simulink model "System3"  (R2025a)
settings: Solver=ode113  StartTime=0.0  StopTime=400  FixedStep=0.01  MaxStep=0.1  RelTol=1e-3
libraries: simulink x3784, slpidlib x2
(part 91 of 160)

== system System3/Battery1/Module3/SubModule_10/Cell9/SOC_Mapping ==
  SOC : Inport
  Cell_Temp : Inport  Port=2
  2-D Lookup Table : Lookup_n-D  LookupTableObject=''  BreakpointsForDimension1Source=Input port  BreakpointsForDimension1=[0 0.1 0.2 0.3 0.4 0.5 0.6 0.7 0.8 0.9 1]  BreakpointsForDimension2=[0 10 20 30 40 50 60]  BreakpointsForDimension1FirstPoint=10  BreakpointsForDimension2FirstPoint=10  BreakpointsForDimension1Spacing=12  BreakpointsForDimension2Spacing=12  IndexSearchMethod=Evenly spaced points  TableSource=Input port  Table=|  InterpMethod=Akima spline  DiagnosticForOutOfRangeInput=Error  InternalRulePriority=Speed  RndMeth=Simplest
      | [
      |     2.954364, 3.109857, 3.273534, 3.3066, 3.34,    3.3734,  3.20473;
      |     3.122427, 3.286765, 3.459753, 3.4947, 3.53,    3.5653,  3.387035;
      |     3.175499, 3.342631, 3.518559, 3.5541, 3.59,    3.6259,  3.444605;
      |     3.210881, 3.379875, 3.557763, 3.5937, 3.63,    3.6663,  3.482985;
      |     3.237417, 3.407808, 3.587166, 3.6234, 3.66,    3.6966,  3.511777;
      |     3.272799, 3.445052, 3.62637,  3.663,  3.7,     3.737,   3.55015;
      |     3.317026, 3.491066, 3.675375, 3.7125, 3.75,    3.7875,  3.598125;
      |     3.387789, 3.566094, 3.753783, 3.7917, 3.83,    3.8683,  3.674885;
      |     3.467398, 3.649892, 3.841992, 3.8808, 3.92,    3.9592,  3.76124;
      |     3.564697, 3.752313, 3.949803, 3.9897, 4.03,    4.0703,  3.866785;
      |     3.653151, 3.845422, 4.047813, 4.0887, 4.13,    4.1713,  3.962735
      | ]
      settings: InputPortMap=u0,u1,p221,p5
  2-D Lookup Table1 : Lookup_n-D  LookupTableObject=''  BreakpointsForDimension1Source=Input port  BreakpointsForDimension1=[0 0.1 0.2 0.3 0.4 0.5 0.6 0.7 0.8 0.9 1]  BreakpointsForDimension2=[0 10 20 30 40 50 60]  BreakpointsForDimension1FirstPoint=10  BreakpointsForDimension2FirstPoint=10  BreakpointsForDimension1Spacing=12  BreakpointsForDimension2Spacing=12  IndexSearchMethod=Evenly spaced points  TableSource=Input port  Table=|  InterpMethod=Akima spline  DiagnosticForOutOfRangeInput=Error  InternalRulePriority=Speed  RndMeth=Simplest
      | [
      |     2.954364, 3.109857, 3.273534, 3.3066, 3.34,    3.3734,  3.20473;
      |     3.122427, 3.286765, 3.459753, 3.4947, 3.53,    3.5653,  3.387035;
      |     3.175499, 3.342631, 3.518559, 3.5541, 3.59,    3.6259,  3.444605;
      |     3.210881, 3.379875, 3.557763, 3.5937, 3.63,    3.6663,  3.482985;
      |     3.237417, 3.407808, 3.587166, 3.6234, 3.66,    3.6966,  3.511777;
      |     3.272799, 3.445052, 3.62637,  3.663,  3.7,     3.737,   3.55015;
      |     3.317026, 3.491066, 3.675375, 3.7125, 3.75,    3.7875,  3.598125;
      |     3.387789, 3.566094, 3.753783, 3.7917, 3.83,    3.8683,  3.674885;
      |     3.467398, 3.649892, 3.841992, 3.8808, 3.92,    3.9592,  3.76124;
      |     3.564697, 3.752313, 3.949803, 3.9897, 4.03,    4.0703,  3.866785;
      |     3.653151, 3.845422, 4.047813, 4.0887, 4.13,    4.1713,  3.962735
      | ]
      settings: InputPortMap=u0,u1,p221,p5
  Lookup Table Dynamic{3..6} (4 alike) : simulink/Lookup Tables/Lookup Table Dynamic  LookUpMeth=Interpolation-Use End Values  OutDataType=fixdt('double')  OutScaling=[]  OutputDataTypeScalingMode=Specify via dialog  OutDataTypeStr=fixdt('double')  DoSatur=off
  Ri : Outport
  R1 : Outport  Port=2
  C1 : Outport  Port=3
  R2 : Outport  Port=4
  C2 : Outport  Port=5
  OCV : Outport  Port=6
  wires:
  SOC/1 -> Lookup Table Dynamic3/1, Lookup Table Dynamic6/1, Lookup Table Dynamic5/1, Lookup Table Dynamic4/1, 2-D Lookup Table1/1, 2-D Lookup Table/1
  [SOC_User] -> 2-D Lookup Table/4, Lookup Table Dynamic6/2, Lookup Table Dynamic5/2, Lookup Table Dynamic4/2, Lookup Table Dynamic3/2, 2-D Lookup Table1/4
  [OCV] -> 2-D Lookup Table/3
  2-D Lookup Table/1 -> OCV/1
  [Ri_User] -> 2-D Lookup Table1/3
  2-D Lookup Table1/1 -> Ri/1
  [R1_User] -> Lookup Table Dynamic3/3
  Lookup Table Dynamic3/1 -> R1/1
  [C1_User] -> Lookup Table Dynamic4/3
  Lookup Table Dynamic4/1 -> C1/1
  [R2_User] -> Lookup Table Dynamic5/3
  Lookup Table Dynamic5/1 -> R2/1
  [C2_User] -> Lookup Table Dynamic6/3
  Lookup Table Dynamic6/1 -> C2/1
  Cell_Temp/1 -> 2-D Lookup Table1/2, 2-D Lookup Table/2

== system System3/Battery1/Module3/SubModule_10/Cell9/Subsystem ==
  Cell_Current : Inport
  Ri : Inport  Port=2
  Add : Sum  Inputs=+-
  Add1 : Sum  Inputs=-+
  Delay : Delay  DelayLength=1  InitialConditionSource=Input port
      settings: InputPortMap=u0,p4
  Divide : Product  Inputs=*/
  From3 : From  TagVisibility=global
  Integrator : Integrator  InitialConditionSource=external
  Product{,1..3} (4 alike) : Product
  Temp_Cell : Outport
  wires:
  Integrator/1 -> Temp_Cell/1, Delay/1
  Cell_Current/1 -> Product/2, Product/1
  Product/1 -> Product1/1
  Ri/1 -> Product1/2
  [h] -> Product2/1
  From3/1 -> Product2/2
  Product2/1 -> Product3/2
  [Temp_ambient] -> Add/2
  Add/1 -> Product3/1
  Product3/1 -> Add1/1
  Product1/1 -> Add1/2
  Add1/1 -> Divide/1
  Divide/1 -> Integrator/1
  [Temp_Iinitial] -> Delay/2, Integrator/2
  Delay/1 -> Add/1
  [Cp] -> Divide/2

== system System3/Battery1/Module3/SubModule_2/Cell1/2RC ==
  Current : Inport
  Ri : Inport  Port=2
  R1 : Inport  Port=3
  C1 : Inport  Port=4
  R2 : Inport  Port=5
  C2 : Inport  Port=6
  RC1 : Subsystem
  RC2 : Subsystem
  Rint : Subsystem
  V1 : Outport
  V2 : Outport  Port=2
  Vi : Outport  Port=3
  wires:
  Current/1 -> Rint/1(Current), RC1/1(Current), RC2/1(Current)
  R1/1 -> RC1/2(R)
  Rint/1(V) -> Vi/1
  C1/1 -> RC1/3(C)
  R2/1 -> RC2/2(R)
  RC1/1(V) -> V1/1
  RC2/1(V) -> V2/1
  C2/1 -> RC2/3(C)
  Ri/1 -> Rint/2(R)

== system System3/Battery1/Module3/SubModule_2/Cell1/SOCEstimator ==
  SOC_Initial : Inport
  Current : Inport  Port=2
  Cell_Capacity : Inport  Port=3
  SOCEstimator : Subsystem
  SOC : Outport
  wires:
  SOCEstimator/1(SOC) -> SOC/1
  SOC_Initial/1 -> SOCEstimator/1(SOC_Initial)
  Current/1 -> SOCEstimator/2(Current)
  Cell_Capacity/1 -> SOCEstimator/3(CellCapacity)

== system System3/Battery1/Module3/SubModule_2/Cell1/SOC_Mapping ==
  SOC : Inport
  Cell_Temp : Inport  Port=2
  2-D Lookup Table : Lookup_n-D  LookupTableObject=''  BreakpointsForDimension1Source=Input port  BreakpointsForDimension1=[0 0.1 0.2 0.3 0.4 0.5 0.6 0.7 0.8 0.9 1]  BreakpointsForDimension2=[0 10 20 30 40 50 60]  BreakpointsForDimension1FirstPoint=10  BreakpointsForDimension2FirstPoint=10  BreakpointsForDimension1Spacing=12  BreakpointsForDimension2Spacing=12  IndexSearchMethod=Evenly spaced points  TableSource=Input port  Table=|  InterpMethod=Akima spline  DiagnosticForOutOfRangeInput=Error  InternalRulePriority=Speed  RndMeth=Simplest
      | [
      |     2.954364, 3.109857, 3.273534, 3.3066, 3.34,    3.3734,  3.20473;
      |     3.122427, 3.286765, 3.459753, 3.4947, 3.53,    3.5653,  3.387035;
      |     3.175499, 3.342631, 3.518559, 3.5541, 3.59,    3.6259,  3.444605;
      |     3.210881, 3.379875, 3.557763, 3.5937, 3.63,    3.6663,  3.482985;
      |     3.237417, 3.407808, 3.587166, 3.6234, 3.66,    3.6966,  3.511777;
      |     3.272799, 3.445052, 3.62637,  3.663,  3.7,     3.737,   3.55015;
      |     3.317026, 3.491066, 3.675375, 3.7125, 3.75,    3.7875,  3.598125;
      |     3.387789, 3.566094, 3.753783, 3.7917, 3.83,    3.8683,  3.674885;
      |     3.467398, 3.649892, 3.841992, 3.8808, 3.92,    3.9592,  3.76124;
      |     3.564697, 3.752313, 3.949803, 3.9897, 4.03,    4.0703,  3.866785;
      |     3.653151, 3.845422, 4.047813, 4.0887, 4.13,    4.1713,  3.962735
      | ]
      settings: InputPortMap=u0,u1,p221,p5
  2-D Lookup Table1 : Lookup_n-D  LookupTableObject=''  BreakpointsForDimension1Source=Input port  BreakpointsForDimension1=[0 0.1 0.2 0.3 0.4 0.5 0.6 0.7 0.8 0.9 1]  BreakpointsForDimension2=[0 10 20 30 40 50 60]  BreakpointsForDimension1FirstPoint=10  BreakpointsForDimension2FirstPoint=10  BreakpointsForDimension1Spacing=12  BreakpointsForDimension2Spacing=12  IndexSearchMethod=Evenly spaced points  TableSource=Input port  Table=|  InterpMethod=Akima spline  DiagnosticForOutOfRangeInput=Error  InternalRulePriority=Speed  RndMeth=Simplest
      | [
      |     2.954364, 3.109857, 3.273534, 3.3066, 3.34,    3.3734,  3.20473;
      |     3.122427, 3.286765, 3.459753, 3.4947, 3.53,    3.5653,  3.387035;
      |     3.175499, 3.342631, 3.518559, 3.5541, 3.59,    3.6259,  3.444605;
      |     3.210881, 3.379875, 3.557763, 3.5937, 3.63,    3.6663,  3.482985;
      |     3.237417, 3.407808, 3.587166, 3.6234, 3.66,    3.6966,  3.511777;
      |     3.272799, 3.445052, 3.62637,  3.663,  3.7,     3.737,   3.55015;
      |     3.317026, 3.491066, 3.675375, 3.7125, 3.75,    3.7875,  3.598125;
      |     3.387789, 3.566094, 3.753783, 3.7917, 3.83,    3.8683,  3.674885;
      |     3.467398, 3.649892, 3.841992, 3.8808, 3.92,    3.9592,  3.76124;
      |     3.564697, 3.752313, 3.949803, 3.9897, 4.03,    4.0703,  3.866785;
      |     3.653151, 3.845422, 4.047813, 4.0887, 4.13,    4.1713,  3.962735
      | ]
      settings: InputPortMap=u0,u1,p221,p5
  Lookup Table Dynamic{3..6} (4 alike) : simulink/Lookup Tables/Lookup Table Dynamic  LookUpMeth=Interpolation-Use End Values  OutDataType=fixdt('double')  OutScaling=[]  OutputDataTypeScalingMode=Specify via dialog  OutDataTypeStr=fixdt('double')  DoSatur=off
  Ri : Outport
  R1 : Outport  Port=2
  C1 : Outport  Port=3
  R2 : Outport  Port=4
  C2 : Outport  Port=5
  OCV : Outport  Port=6
  wires:
  SOC/1 -> Lookup Table Dynamic3/1, Lookup Table Dynamic6/1, Lookup Table Dynamic5/1, Lookup Table Dynamic4/1, 2-D Lookup Table1/1, 2-D Lookup Table/1
  [SOC_User] -> 2-D Lookup Table/4, Lookup Table Dynamic6/2, Lookup Table Dynamic5/2, Lookup Table Dynamic4/2, Lookup Table Dynamic3/2, 2-D Lookup Table1/4
  [OCV] -> 2-D Lookup Table/3
  2-D Lookup Table/1 -> OCV/1
  [Ri_User] -> 2-D Lookup Table1/3
  2-D Lookup Table1/1 -> Ri/1
  [R1_User] -> Lookup Table Dynamic3/3
  Lookup Table Dynamic3/1 -> R1/1
  [C1_User] -> Lookup Table Dynamic4/3
  Lookup Table Dynamic4/1 -> C1/1
  [R2_User] -> Lookup Table Dynamic5/3
  Lookup Table Dynamic5/1 -> R2/1
  [C2_User] -> Lookup Table Dynamic6/3
  Lookup Table Dynamic6/1 -> C2/1
  Cell_Temp/1 -> 2-D Lookup Table1/2, 2-D Lookup Table/2

== system System3/Battery1/Module3/SubModule_2/Cell1/Subsystem ==
  Cell_Current : Inport
  Ri : Inport  Port=2
  Add : Sum  Inputs=+-
  Add1 : Sum  Inputs=-+
  Delay : Delay  DelayLength=1  InitialConditionSource=Input port
      settings: InputPortMap=u0,p4
  Divide : Product  Inputs=*/
  From3 : From  TagVisibility=global
  Integrator : Integrator  InitialConditionSource=external
  Product{,1..3} (4 alike) : Product
  Temp_Cell : Outport
  wires:
  Integrator/1 -> Temp_Cell/1, Delay/1
  Cell_Current/1 -> Product/2, Product/1
  Product/1 -> Product1/1
  Ri/1 -> Product1/2
  [h] -> Product2/1
  From3/1 -> Product2/2
  Product2/1 -> Product3/2
  [Temp_ambient] -> Add/2
  Add/1 -> Product3/1
  Product3/1 -> Add1/1
  Product1/1 -> Add1/2
  Add1/1 -> Divide/1
  Divide/1 -> Integrator/1
  [Temp_Iinitial] -> Delay/2, Integrator/2
  Delay/1 -> Add/1
  [Cp] -> Divide/2

== system System3/Battery1/Module3/SubModule_2/Cell10/2RC ==
  Current : Inport
  Ri : Inport  Port=2
  R1 : Inport  Port=3
  C1 : Inport  Port=4
  R2 : Inport  Port=5
  C2 : Inport  Port=6
  RC1 : Subsystem
  RC2 : Subsystem
  Rint : Subsystem
  V1 : Outport
  V2 : Outport  Port=2
  Vi : Outport  Port=3
  wires:
  Current/1 -> Rint/1(Current), RC1/1(Current), RC2/1(Current)
  R1/1 -> RC1/2(R)
  Rint/1(V) -> Vi/1
  C1/1 -> RC1/3(C)
  R2/1 -> RC2/2(R)
  RC1/1(V) -> V1/1
  RC2/1(V) -> V2/1
  C2/1 -> RC2/3(C)
  Ri/1 -> Rint/2(R)

== system System3/Battery1/Module3/SubModule_2/Cell10/SOCEstimator ==
  SOC_Initial : Inport
  Current : Inport  Port=2
  Cell_Capacity : Inport  Port=3
  SOCEstimator : Subsystem
  SOC : Outport
  wires:
  SOCEstimator/1(SOC) -> SOC/1
  SOC_Initial/1 -> SOCEstimator/1(SOC_Initial)
  Current/1 -> SOCEstimator/2(Current)
  Cell_Capacity/1 -> SOCEstimator/3(CellCapacity)

== system System3/Battery1/Module3/SubModule_2/Cell10/SOC_Mapping ==
  SOC : Inport
  Cell_Temp : Inport  Port=2
  2-D Lookup Table : Lookup_n-D  LookupTableObject=''  BreakpointsForDimension1Source=Input port  BreakpointsForDimension1=[0 0.1 0.2 0.3 0.4 0.5 0.6 0.7 0.8 0.9 1]  BreakpointsForDimension2=[0 10 20 30 40 50 60]  BreakpointsForDimension1FirstPoint=10  BreakpointsForDimension2FirstPoint=10  BreakpointsForDimension1Spacing=12  BreakpointsForDimension2Spacing=12  IndexSearchMethod=Evenly spaced points  TableSource=Input port  Table=|  InterpMethod=Akima spline  DiagnosticForOutOfRangeInput=Error  InternalRulePriority=Speed  RndMeth=Simplest
      | [
      |     2.954364, 3.109857, 3.273534, 3.3066, 3.34,    3.3734,  3.20473;
      |     3.122427, 3.286765, 3.459753, 3.4947, 3.53,    3.5653,  3.387035;
      |     3.175499, 3.342631, 3.518559, 3.5541, 3.59,    3.6259,  3.444605;
      |     3.210881, 3.379875, 3.557763, 3.5937, 3.63,    3.6663,  3.482985;
      |     3.237417, 3.407808, 3.587166, 3.6234, 3.66,    3.6966,  3.511777;
      |     3.272799, 3.445052, 3.62637,  3.663,  3.7,     3.737,   3.55015;
      |     3.317026, 3.491066, 3.675375, 3.7125, 3.75,    3.7875,  3.598125;
      |     3.387789, 3.566094, 3.753783, 3.7917, 3.83,    3.8683,  3.674885;
      |     3.467398, 3.649892, 3.841992, 3.8808, 3.92,    3.9592,  3.76124;
      |     3.564697, 3.752313, 3.949803, 3.9897, 4.03,    4.0703,  3.866785;
      |     3.653151, 3.845422, 4.047813, 4.0887, 4.13,    4.1713,  3.962735
      | ]
      settings: InputPortMap=u0,u1,p221,p5
  2-D Lookup Table1 : Lookup_n-D  LookupTableObject=''  BreakpointsForDimension1Source=Input port  BreakpointsForDimension1=[0 0.1 0.2 0.3 0.4 0.5 0.6 0.7 0.8 0.9 1]  BreakpointsForDimension2=[0 10 20 30 40 50 60]  BreakpointsForDimension1FirstPoint=10  BreakpointsForDimension2FirstPoint=10  BreakpointsForDimension1Spacing=12  BreakpointsForDimension2Spacing=12  IndexSearchMethod=Evenly spaced points  TableSource=Input port  Table=|  InterpMethod=Akima spline  DiagnosticForOutOfRangeInput=Error  InternalRulePriority=Speed  RndMeth=Simplest
      | [
      |     2.954364, 3.109857, 3.273534, 3.3066, 3.34,    3.3734,  3.20473;
      |     3.122427, 3.286765, 3.459753, 3.4947, 3.53,    3.5653,  3.387035;
      |     3.175499, 3.342631, 3.518559, 3.5541, 3.59,    3.6259,  3.444605;
      |     3.210881, 3.379875, 3.557763, 3.5937, 3.63,    3.6663,  3.482985;
      |     3.237417, 3.407808, 3.587166, 3.6234, 3.66,    3.6966,  3.511777;
      |     3.272799, 3.445052, 3.62637,  3.663,  3.7,     3.737,   3.55015;
      |     3.317026, 3.491066, 3.675375, 3.7125, 3.75,    3.7875,  3.598125;
      |     3.387789, 3.566094, 3.753783, 3.7917, 3.83,    3.8683,  3.674885;
      |     3.467398, 3.649892, 3.841992, 3.8808, 3.92,    3.9592,  3.76124;
      |     3.564697, 3.752313, 3.949803, 3.9897, 4.03,    4.0703,  3.866785;
      |     3.653151, 3.845422, 4.047813, 4.0887, 4.13,    4.1713,  3.962735
      | ]
      settings: InputPortMap=u0,u1,p221,p5
  Lookup Table Dynamic{3..6} (4 alike) : simulink/Lookup Tables/Lookup Table Dynamic  LookUpMeth=Interpolation-Use End Values  OutDataType=fixdt('double')  OutScaling=[]  OutputDataTypeScalingMode=Specify via dialog  OutDataTypeStr=fixdt('double')  DoSatur=off
  Ri : Outport
  R1 : Outport  Port=2
  C1 : Outport  Port=3
  R2 : Outport  Port=4
  C2 : Outport  Port=5
  OCV : Outport  Port=6
  wires:
  SOC/1 -> Lookup Table Dynamic3/1, Lookup Table Dynamic6/1, Lookup Table Dynamic5/1, Lookup Table Dynamic4/1, 2-D Lookup Table1/1, 2-D Lookup Table/1
  [SOC_User] -> 2-D Lookup Table/4, Lookup Table Dynamic6/2, Lookup Table Dynamic5/2, Lookup Table Dynamic4/2, Lookup Table Dynamic3/2, 2-D Lookup Table1/4
  [OCV] -> 2-D Lookup Table/3
  2-D Lookup Table/1 -> OCV/1
  [Ri_User] -> 2-D Lookup Table1/3
  2-D Lookup Table1/1 -> Ri/1
  [R1_User] -> Lookup Table Dynamic3/3
  Lookup Table Dynamic3/1 -> R1/1
  [C1_User] -> Lookup Table Dynamic4/3
  Lookup Table Dynamic4/1 -> C1/1
  [R2_User] -> Lookup Table Dynamic5/3
  Lookup Table Dynamic5/1 -> R2/1
  [C2_User] -> Lookup Table Dynamic6/3
  Lookup Table Dynamic6/1 -> C2/1
  Cell_Temp/1 -> 2-D Lookup Table1/2, 2-D Lookup Table/2

== system System3/Battery1/Module3/SubModule_2/Cell10/Subsystem ==
  Cell_Current : Inport
  Ri : Inport  Port=2
  Add : Sum  Inputs=+-
  Add1 : Sum  Inputs=-+
  Delay : Delay  DelayLength=1  InitialConditionSource=Input port
      settings: InputPortMap=u0,p4
  Divide : Product  Inputs=*/
  From3 : From  TagVisibility=global
  Integrator : Integrator  InitialConditionSource=external
  Product{,1..3} (4 alike) : Product
  Temp_Cell : Outport
  wires:
  Integrator/1 -> Temp_Cell/1, Delay/1
  Cell_Current/1 -> Product/2, Product/1
  Product/1 -> Product1/1
  Ri/1 -> Product1/2
  [h] -> Product2/1
  From3/1 -> Product2/2
  Product2/1 -> Product3/2
  [Temp_ambient] -> Add/2
  Add/1 -> Product3/1
  Product3/1 -> Add1/1
  Product1/1 -> Add1/2
  Add1/1 -> Divide/1
  Divide/1 -> Integrator/1
  [Temp_Iinitial] -> Delay/2, Integrator/2
  Delay/1 -> Add/1
  [Cp] -> Divide/2

== system System3/Battery1/Module3/SubModule_2/Cell11/2RC ==
  Current : Inport
  Ri : Inport  Port=2
  R1 : Inport  Port=3
  C1 : Inport  Port=4
  R2 : Inport  Port=5
  C2 : Inport  Port=6
  RC1 : Subsystem
  RC2 : Subsystem
  Rint : Subsystem
  V1 : Outport
  V2 : Outport  Port=2
  Vi : Outport  Port=3
  wires:
  Ri/1 -> Rint/2(R)
  C2/1 -> RC2/3(C)
  RC2/1(V) -> V2/1
  RC1/1(V) -> V1/1
  R2/1 -> RC2/2(R)
  C1/1 -> RC1/3(C)
  Rint/1(V) -> Vi/1
  R1/1 -> RC1/2(R)
  Current/1 -> RC2/1(Current), RC1/1(Current), Rint/1(Current)

== system System3/Battery1/Module3/SubModule_2/Cell11/SOCEstimator ==
  SOC_Initial : Inport
  Current : Inport  Port=2
  Cell_Capacity : Inport  Port=3
  SOCEstimator : Subsystem
  SOC : Outport
  wires:
  Cell_Capacity/1 -> SOCEstimator/3(CellCapacity)
  Current/1 -> SOCEstimator/2(Current)
  SOC_Initial/1 -> SOCEstimator/1(SOC_Initial)
  SOCEstimator/1(SOC) -> SOC/1

== system System3/Battery1/Module3/SubModule_2/Cell11/SOC_Mapping ==
  SOC : Inport
  Cell_Temp : Inport  Port=2
  2-D Lookup Table : Lookup_n-D  LookupTableObject=''  BreakpointsForDimension1Source=Input port  BreakpointsForDimension1=[0 0.1 0.2 0.3 0.4 0.5 0.6 0.7 0.8 0.9 1]  BreakpointsForDimension2=[0 10 20 30 40 50 60]  BreakpointsForDimension1FirstPoint=10  BreakpointsForDimension2FirstPoint=10  BreakpointsForDimension1Spacing=12  BreakpointsForDimension2Spacing=12  IndexSearchMethod=Evenly spaced points  TableSource=Input port  Table=|  InterpMethod=Akima spline  DiagnosticForOutOfRangeInput=Error  InternalRulePriority=Speed  RndMeth=Simplest
      | [
      |     2.954364, 3.109857, 3.273534, 3.3066, 3.34,    3.3734,  3.20473;
      |     3.122427, 3.286765, 3.459753, 3.4947, 3.53,    3.5653,  3.387035;
      |     3.175499, 3.342631, 3.518559, 3.5541, 3.59,    3.6259,  3.444605;
      |     3.210881, 3.379875, 3.557763, 3.5937, 3.63,    3.6663,  3.482985;
      |     3.237417, 3.407808, 3.587166, 3.6234, 3.66,    3.6966,  3.511777;
      |     3.272799, 3.445052, 3.62637,  3.663,  3.7,     3.737,   3.55015;
      |     3.317026, 3.491066, 3.675375, 3.7125, 3.75,    3.7875,  3.598125;
      |     3.387789, 3.566094, 3.753783, 3.7917, 3.83,    3.8683,  3.674885;
      |     3.467398, 3.649892, 3.841992, 3.8808, 3.92,    3.9592,  3.76124;
      |     3.564697, 3.752313, 3.949803, 3.9897, 4.03,    4.0703,  3.866785;
      |     3.653151, 3.845422, 4.047813, 4.0887, 4.13,    4.1713,  3.962735
      | ]
      settings: InputPortMap=u0,u1,p221,p5
  2-D Lookup Table1 : Lookup_n-D  LookupTableObject=''  BreakpointsForDimension1Source=Input port  BreakpointsForDimension1=[0 0.1 0.2 0.3 0.4 0.5 0.6 0.7 0.8 0.9 1]  BreakpointsForDimension2=[0 10 20 30 40 50 60]  BreakpointsForDimension1FirstPoint=10  BreakpointsForDimension2FirstPoint=10  BreakpointsForDimension1Spacing=12  BreakpointsForDimension2Spacing=12  IndexSearchMethod=Evenly spaced points  TableSource=Input port  Table=|  InterpMethod=Akima spline  DiagnosticForOutOfRangeInput=Error  InternalRulePriority=Speed  RndMeth=Simplest
      | [
      |     2.954364, 3.109857, 3.273534, 3.3066, 3.34,    3.3734,  3.20473;
      |     3.122427, 3.286765, 3.459753, 3.4947, 3.53,    3.5653,  3.387035;
      |     3.175499, 3.342631, 3.518559, 3.5541, 3.59,    3.6259,  3.444605;
      |     3.210881, 3.379875, 3.557763, 3.5937, 3.63,    3.6663,  3.482985;
      |     3.237417, 3.407808, 3.587166, 3.6234, 3.66,    3.6966,  3.511777;
      |     3.272799, 3.445052, 3.62637,  3.663,  3.7,     3.737,   3.55015;
      |     3.317026, 3.491066, 3.675375, 3.7125, 3.75,    3.7875,  3.598125;
      |     3.387789, 3.566094, 3.753783, 3.7917, 3.83,    3.8683,  3.674885;
      |     3.467398, 3.649892, 3.841992, 3.8808, 3.92,    3.9592,  3.76124;
      |     3.564697, 3.752313, 3.949803, 3.9897, 4.03,    4.0703,  3.866785;
      |     3.653151, 3.845422, 4.047813, 4.0887, 4.13,    4.1713,  3.962735
      | ]
      settings: InputPortMap=u0,u1,p221,p5
  Lookup Table Dynamic{3..6} (4 alike) : simulink/Lookup Tables/Lookup Table Dynamic  LookUpMeth=Interpolation-Use End Values  OutDataType=fixdt('double')  OutScaling=[]  OutputDataTypeScalingMode=Specify via dialog  OutDataTypeStr=fixdt('double')  DoSatur=off
  Ri : Outport
  R1 : Outport  Port=2
  C1 : Outport  Port=3
  R2 : Outport  Port=4
  C2 : Outport  Port=5
  OCV : Outport  Port=6
  wires:
  Cell_Temp/1 -> 2-D Lookup Table/2, 2-D Lookup Table1/2
  Lookup Table Dynamic6/1 -> C2/1
  [C2_User] -> Lookup Table Dynamic6/3
  Lookup Table Dynamic5/1 -> R2/1
  [R2_User] -> Lookup Table Dynamic5/3
  Lookup Table Dynamic4/1 -> C1/1
  [C1_User] -> Lookup Table Dynamic4/3
  Lookup Table Dynamic3/1 -> R1/1
  [R1_User] -> Lookup Table Dynamic3/3
  2-D Lookup Table1/1 -> Ri/1
  [Ri_User] -> 2-D Lookup Table1/3
  2-D Lookup Table/1 -> OCV/1
  [OCV] -> 2-D Lookup Table/3
  [SOC_User] -> 2-D Lookup Table1/4, Lookup Table Dynamic3/2, Lookup Table Dynamic4/2, Lookup Table Dynamic5/2, Lookup Table Dynamic6/2, 2-D Lookup Table/4
  SOC/1 -> 2-D Lookup Table/1, 2-D Lookup Table1/1, Lookup Table Dynamic4/1, Lookup Table Dynamic5/1, Lookup Table Dynamic6/1, Lookup Table Dynamic3/1

== system System3/Battery1/Module3/SubModule_2/Cell11/Subsystem ==
  Cell_Current : Inport
  Ri : Inport  Port=2
  Add : Sum  Inputs=+-
  Add1 : Sum  Inputs=-+
  Delay : Delay  DelayLength=1  InitialConditionSource=Input port
      settings: InputPortMap=u0,p4
  Divide : Product  Inputs=*/
  From3 : From  TagVisibility=global
  Integrator : Integrator  InitialConditionSource=external
  Product{,1..3} (4 alike) : Product
  Temp_Cell : Outport
  wires:
  [Cp] -> Divide/2
  Delay/1 -> Add/1
  [Temp_Iinitial] -> Integrator/2, Delay/2
  Divide/1 -> Integrator/1
  Add1/1 -> Divide/1
  Product1/1 -> Add1/2
  Product3/1 -> Add1/1
  Add/1 -> Product3/1
  [Temp_ambient] -> Add/2
  Product2/1 -> Product3/2
  From3/1 -> Product2/2
  [h] -> Product2/1
  Ri/1 -> Product1/2
  Product/1 -> Product1/1
  Cell_Current/1 -> Product/1, Product/2
  Integrator/1 -> Delay/1, Temp_Cell/1

== system System3/Battery1/Module3/SubModule_2/Cell12/2RC ==
  Current : Inport
  Ri : Inport  Port=2
  R1 : Inport  Port=3
  C1 : Inport  Port=4
  R2 : Inport  Port=5
  C2 : Inport  Port=6
  RC1 : Subsystem
  RC2 : Subsystem
  Rint : Subsystem
  V1 : Outport
  V2 : Outport  Port=2
  Vi : Outport  Port=3
  wires:
  Current/1 -> Rint/1(Current), RC1/1(Current), RC2/1(Current)
  R1/1 -> RC1/2(R)
  Rint/1(V) -> Vi/1
  C1/1 -> RC1/3(C)
  R2/1 -> RC2/2(R)
  RC1/1(V) -> V1/1
  RC2/1(V) -> V2/1
  C2/1 -> RC2/3(C)
  Ri/1 -> Rint/2(R)

== system System3/Battery1/Module3/SubModule_2/Cell12/SOCEstimator ==
  SOC_Initial : Inport
  Current : Inport  Port=2
  Cell_Capacity : Inport  Port=3
  SOCEstimator : Subsystem
  SOC : Outport
  wires:
  SOCEstimator/1(SOC) -> SOC/1
  SOC_Initial/1 -> SOCEstimator/1(SOC_Initial)
  Current/1 -> SOCEstimator/2(Current)
  Cell_Capacity/1 -> SOCEstimator/3(CellCapacity)

== system System3/Battery1/Module3/SubModule_2/Cell12/SOC_Mapping ==
  SOC : Inport
  Cell_Temp : Inport  Port=2
  2-D Lookup Table : Lookup_n-D  LookupTableObject=''  BreakpointsForDimension1Source=Input port  BreakpointsForDimension1=[0 0.1 0.2 0.3 0.4 0.5 0.6 0.7 0.8 0.9 1]  BreakpointsForDimension2=[0 10 20 30 40 50 60]  BreakpointsForDimension1FirstPoint=10  BreakpointsForDimension2FirstPoint=10  BreakpointsForDimension1Spacing=12  BreakpointsForDimension2Spacing=12  IndexSearchMethod=Evenly spaced points  TableSource=Input port  Table=|  InterpMethod=Akima spline  DiagnosticForOutOfRangeInput=Error  InternalRulePriority=Speed  RndMeth=Simplest
      | [
      |     2.954364, 3.109857, 3.273534, 3.3066, 3.34,    3.3734,  3.20473;
      |     3.122427, 3.286765, 3.459753, 3.4947, 3.53,    3.5653,  3.387035;
      |     3.175499, 3.342631, 3.518559, 3.5541, 3.59,    3.6259,  3.444605;
      |     3.210881, 3.379875, 3.557763, 3.5937, 3.63,    3.6663,  3.482985;
      |     3.237417, 3.407808, 3.587166, 3.6234, 3.66,    3.6966,  3.511777;
      |     3.272799, 3.445052, 3.62637,  3.663,  3.7,     3.737,   3.55015;
      |     3.317026, 3.491066, 3.675375, 3.7125, 3.75,    3.7875,  3.598125;
      |     3.387789, 3.566094, 3.753783, 3.7917, 3.83,    3.8683,  3.674885;
      |     3.467398, 3.649892, 3.841992, 3.8808, 3.92,    3.9592,  3.76124;
      |     3.564697, 3.752313, 3.949803, 3.9897, 4.03,    4.0703,  3.866785;
      |     3.653151, 3.845422, 4.047813, 4.0887, 4.13,    4.1713,  3.962735
      | ]
      settings: InputPortMap=u0,u1,p221,p5
  2-D Lookup Table1 : Lookup_n-D  LookupTableObject=''  BreakpointsForDimension1Source=Input port  BreakpointsForDimension1=[0 0.1 0.2 0.3 0.4 0.5 0.6 0.7 0.8 0.9 1]  BreakpointsForDimension2=[0 10 20 30 40 50 60]  BreakpointsForDimension1FirstPoint=10  BreakpointsForDimension2FirstPoint=10  BreakpointsForDimension1Spacing=12  BreakpointsForDimension2Spacing=12  IndexSearchMethod=Evenly spaced points  TableSource=Input port  Table=|  InterpMethod=Akima spline  DiagnosticForOutOfRangeInput=Error  InternalRulePriority=Speed  RndMeth=Simplest
      | [
      |     2.954364, 3.109857, 3.273534, 3.3066, 3.34,    3.3734,  3.20473;
      |     3.122427, 3.286765, 3.459753, 3.4947, 3.53,    3.5653,  3.387035;
      |     3.175499, 3.342631, 3.518559, 3.5541, 3.59,    3.6259,  3.444605;
      |     3.210881, 3.379875, 3.557763, 3.5937, 3.63,    3.6663,  3.482985;
      |     3.237417, 3.407808, 3.587166, 3.6234, 3.66,    3.6966,  3.511777;
      |     3.272799, 3.445052, 3.62637,  3.663,  3.7,     3.737,   3.55015;
      |     3.317026, 3.491066, 3.675375, 3.7125, 3.75,    3.7875,  3.598125;
      |     3.387789, 3.566094, 3.753783, 3.7917, 3.83,    3.8683,  3.674885;
      |     3.467398, 3.649892, 3.841992, 3.8808, 3.92,    3.9592,  3.76124;
      |     3.564697, 3.752313, 3.949803, 3.9897, 4.03,    4.0703,  3.866785;
      |     3.653151, 3.845422, 4.047813, 4.0887, 4.13,    4.1713,  3.962735
      | ]
      settings: InputPortMap=u0,u1,p221,p5
  Lookup Table Dynamic{3..6} (4 alike) : simulink/Lookup Tables/Lookup Table Dynamic  LookUpMeth=Interpolation-Use End Values  OutDataType=fixdt('double')  OutScaling=[]  OutputDataTypeScalingMode=Specify via dialog  OutDataTypeStr=fixdt('double')  DoSatur=off
  Ri : Outport
  R1 : Outport  Port=2
  C1 : Outport  Port=3
  R2 : Outport  Port=4
  C2 : Outport  Port=5
  OCV : Outport  Port=6
  wires:
  SOC/1 -> Lookup Table Dynamic3/1, Lookup Table Dynamic6/1, Lookup Table Dynamic5/1, Lookup Table Dynamic4/1, 2-D Lookup Table1/1, 2-D Lookup Table/1
  [SOC_User] -> 2-D Lookup Table/4, Lookup Table Dynamic6/2, Lookup Table Dynamic5/2, Lookup Table Dynamic4/2, Lookup Table Dynamic3/2, 2-D Lookup Table1/4
  [OCV] -> 2-D Lookup Table/3
  2-D Lookup Table/1 -> OCV/1
  [Ri_User] -> 2-D Lookup Table1/3
  2-D Lookup Table1/1 -> Ri/1
  [R1_User] -> Lookup Table Dynamic3/3
  Lookup Table Dynamic3/1 -> R1/1
  [C1_User] -> Lookup Table Dynamic4/3
  Lookup Table Dynamic4/1 -> C1/1
  [R2_User] -> Lookup Table Dynamic5/3
  Lookup Table Dynamic5/1 -> R2/1
  [C2_User] -> Lookup Table Dynamic6/3
  Lookup Table Dynamic6/1 -> C2/1
  Cell_Temp/1 -> 2-D Lookup Table1/2, 2-D Lookup Table/2

== system System3/Battery1/Module3/SubModule_2/Cell12/Subsystem ==
  Cell_Current : Inport
  Ri : Inport  Port=2
  Add : Sum  Inputs=+-
  Add1 : Sum  Inputs=-+
  Delay : Delay  DelayLength=1  InitialConditionSource=Input port
      settings: InputPortMap=u0,p4
  Divide : Product  Inputs=*/
  From3 : From  TagVisibility=global
  Integrator : Integrator  InitialConditionSource=external
  Product{,1..3} (4 alike) : Product
  Temp_Cell : Outport
  wires:
  Integrator/1 -> Temp_Cell/1, Delay/1
  Cell_Current/1 -> Product/2, Product/1
  Product/1 -> Product1/1
  Ri/1 -> Product1/2
  [h] -> Product2/1
  From3/1 -> Product2/2
  Product2/1 -> Product3/2
  [Temp_ambient] -> Add/2
  Add/1 -> Product3/1
  Product3/1 -> Add1/1
  Product1/1 -> Add1/2
  Add1/1 -> Divide/1
  Divide/1 -> Integrator/1
  [Temp_Iinitial] -> Delay/2, Integrator/2
  Delay/1 -> Add/1
  [Cp] -> Divide/2

== system System3/Battery1/Module3/SubModule_2/Cell13/2RC ==
  Current : Inport
  Ri : Inport  Port=2
  R1 : Inport  Port=3
  C1 : Inport  Port=4
  R2 : Inport  Port=5
  C2 : Inport  Port=6
  RC1 : Subsystem
  RC2 : Subsystem
  Rint : Subsystem
  V1 : Outport
  V2 : Outport  Port=2
  Vi : Outport  Port=3
  wires:
  Ri/1 -> Rint/2(R)
  C2/1 -> RC2/3(C)
  RC2/1(V) -> V2/1
  RC1/1(V) -> V1/1
  R2/1 -> RC2/2(R)
  C1/1 -> RC1/3(C)
  Rint/1(V) -> Vi/1
  R1/1 -> RC1/2(R)
  Current/1 -> RC2/1(Current), RC1/1(Current), Rint/1(Current)

== system System3/Battery1/Module3/SubModule_2/Cell13/SOCEstimator ==
  SOC_Initial : Inport
  Current : Inport  Port=2
  Cell_Capacity : Inport  Port=3
  SOCEstimator : Subsystem
  SOC : Outport
  wires:
  Cell_Capacity/1 -> SOCEstimator/3(CellCapacity)
  Current/1 -> SOCEstimator/2(Current)
  SOC_Initial/1 -> SOCEstimator/1(SOC_Initial)
  SOCEstimator/1(SOC) -> SOC/1

== system System3/Battery1/Module3/SubModule_2/Cell13/SOC_Mapping ==
  SOC : Inport
  Cell_Temp : Inport  Port=2
  2-D Lookup Table : Lookup_n-D  LookupTableObject=''  BreakpointsForDimension1Source=Input port  BreakpointsForDimension1=[0 0.1 0.2 0.3 0.4 0.5 0.6 0.7 0.8 0.9 1]  BreakpointsForDimension2=[0 10 20 30 40 50 60]  BreakpointsForDimension1FirstPoint=10  BreakpointsForDimension2FirstPoint=10  BreakpointsForDimension1Spacing=12  BreakpointsForDimension2Spacing=12  IndexSearchMethod=Evenly spaced points  TableSource=Input port  Table=|  InterpMethod=Akima spline  DiagnosticForOutOfRangeInput=Error  InternalRulePriority=Speed  RndMeth=Simplest
      | [
      |     2.954364, 3.109857, 3.273534, 3.3066, 3.34,    3.3734,  3.20473;
      |     3.122427, 3.286765, 3.459753, 3.4947, 3.53,    3.5653,  3.387035;
      |     3.175499, 3.342631, 3.518559, 3.5541, 3.59,    3.6259,  3.444605;
      |     3.210881, 3.379875, 3.557763, 3.5937, 3.63,    3.6663,  3.482985;
      |     3.237417, 3.407808, 3.587166, 3.6234, 3.66,    3.6966,  3.511777;
      |     3.272799, 3.445052, 3.62637,  3.663,  3.7,     3.737,   3.55015;
      |     3.317026, 3.491066, 3.675375, 3.7125, 3.75,    3.7875,  3.598125;
      |     3.387789, 3.566094, 3.753783, 3.7917, 3.83,    3.8683,  3.674885;
      |     3.467398, 3.649892, 3.841992, 3.8808, 3.92,    3.9592,  3.76124;
      |     3.564697, 3.752313, 3.949803, 3.9897, 4.03,    4.0703,  3.866785;
      |     3.653151, 3.845422, 4.047813, 4.0887, 4.13,    4.1713,  3.962735
      | ]
      settings: InputPortMap=u0,u1,p221,p5
  2-D Lookup Table1 : Lookup_n-D  LookupTableObject=''  BreakpointsForDimension1Source=Input port  BreakpointsForDimension1=[0 0.1 0.2 0.3 0.4 0.5 0.6 0.7 0.8 0.9 1]  BreakpointsForDimension2=[0 10 20 30 40 50 60]  BreakpointsForDimension1FirstPoint=10  BreakpointsForDimension2FirstPoint=10  BreakpointsForDimension1Spacing=12  BreakpointsForDimension2Spacing=12  IndexSearchMethod=Evenly spaced points  TableSource=Input port  Table=|  InterpMethod=Akima spline  DiagnosticForOutOfRangeInput=Error  InternalRulePriority=Speed  RndMeth=Simplest
      | [
      |     2.954364, 3.109857, 3.273534, 3.3066, 3.34,    3.3734,  3.20473;
      |     3.122427, 3.286765, 3.459753, 3.4947, 3.53,    3.5653,  3.387035;
      |     3.175499, 3.342631, 3.518559, 3.5541, 3.59,    3.6259,  3.444605;
      |     3.210881, 3.379875, 3.557763, 3.5937, 3.63,    3.6663,  3.482985;
      |     3.237417, 3.407808, 3.587166, 3.6234, 3.66,    3.6966,  3.511777;
      |     3.272799, 3.445052, 3.62637,  3.663,  3.7,     3.737,   3.55015;
      |     3.317026, 3.491066, 3.675375, 3.7125, 3.75,    3.7875,  3.598125;
      |     3.387789, 3.566094, 3.753783, 3.7917, 3.83,    3.8683,  3.674885;
      |     3.467398, 3.649892, 3.841992, 3.8808, 3.92,    3.9592,  3.76124;
      |     3.564697, 3.752313, 3.949803, 3.9897, 4.03,    4.0703,  3.866785;
      |     3.653151, 3.845422, 4.047813, 4.0887, 4.13,    4.1713,  3.962735
      | ]
      settings: InputPortMap=u0,u1,p221,p5
  Lookup Table Dynamic{3..6} (4 alike) : simulink/Lookup Tables/Lookup Table Dynamic  LookUpMeth=Interpolation-Use End Values  OutDataType=fixdt('double')  OutScaling=[]  OutputDataTypeScalingMode=Specify via dialog  OutDataTypeStr=fixdt('double')  DoSatur=off
  Ri : Outport
  R1 : Outport  Port=2
  C1 : Outport  Port=3
  R2 : Outport  Port=4
  C2 : Outport  Port=5
  OCV : Outport  Port=6
  wires:
  Cell_Temp/1 -> 2-D Lookup Table/2, 2-D Lookup Table1/2
  Lookup Table Dynamic6/1 -> C2/1
  [C2_User] -> Lookup Table Dynamic6/3
  Lookup Table Dynamic5/1 -> R2/1
  [R2_User] -> Lookup Table Dynamic5/3
  Lookup Table Dynamic4/1 -> C1/1
  [C1_User] -> Lookup Table Dynamic4/3
  Lookup Table Dynamic3/1 -> R1/1
  [R1_User] -> Lookup Table Dynamic3/3
  2-D Lookup Table1/1 -> Ri/1
  [Ri_User] -> 2-D Lookup Table1/3
  2-D Lookup Table/1 -> OCV/1
  [OCV] -> 2-D Lookup Table/3
  [SOC_User] -> 2-D Lookup Table1/4, Lookup Table Dynamic3/2, Lookup Table Dynamic4/2, Lookup Table Dynamic5/2, Lookup Table Dynamic6/2, 2-D Lookup Table/4
  SOC/1 -> 2-D Lookup Table/1, 2-D Lookup Table1/1, Lookup Table Dynamic4/1, Lookup Table Dynamic5/1, Lookup Table Dynamic6/1, Lookup Table Dynamic3/1

== system System3/Battery1/Module3/SubModule_2/Cell13/Subsystem ==
  Cell_Current : Inport
  Ri : Inport  Port=2
  Add : Sum  Inputs=+-
  Add1 : Sum  Inputs=-+
  Delay : Delay  DelayLength=1  InitialConditionSource=Input port
      settings: InputPortMap=u0,p4
  Divide : Product  Inputs=*/
  From3 : From  TagVisibility=global
  Integrator : Integrator  InitialConditionSource=external
  Product{,1..3} (4 alike) : Product
  Temp_Cell : Outport
  wires:
  [Cp] -> Divide/2
  Delay/1 -> Add/1
  [Temp_Iinitial] -> Integrator/2, Delay/2
  Divide/1 -> Integrator/1
  Add1/1 -> Divide/1
  Product1/1 -> Add1/2
  Product3/1 -> Add1/1
  Add/1 -> Product3/1
  [Temp_ambient] -> Add/2
  Product2/1 -> Product3/2
  From3/1 -> Product2/2
  [h] -> Product2/1
  Ri/1 -> Product1/2
  Product/1 -> Product1/1
  Cell_Current/1 -> Product/1, Product/2
  Integrator/1 -> Delay/1, Temp_Cell/1

== system System3/Battery1/Module3/SubModule_2/Cell14/2RC ==
  Current : Inport
  Ri : Inport  Port=2
  R1 : Inport  Port=3
  C1 : Inport  Port=4
  R2 : Inport  Port=5
  C2 : Inport  Port=6
  RC1 : Subsystem
  RC2 : Subsystem
  Rint : Subsystem
  V1 : Outport
  V2 : Outport  Port=2
  Vi : Outport  Port=3
  wires:
  Ri/1 -> Rint/2(R)
  C2/1 -> RC2/3(C)
  RC2/1(V) -> V2/1
  RC1/1(V) -> V1/1
  R2/1 -> RC2/2(R)
  C1/1 -> RC1/3(C)
  Rint/1(V) -> Vi/1
  R1/1 -> RC1/2(R)
  Current/1 -> RC2/1(Current), RC1/1(Current), Rint/1(Current)

== system System3/Battery1/Module3/SubModule_2/Cell14/SOCEstimator ==
  SOC_Initial : Inport
  Current : Inport  Port=2
  Cell_Capacity : Inport  Port=3
  SOCEstimator : Subsystem
  SOC : Outport
  wires:
  Cell_Capacity/1 -> SOCEstimator/3(CellCapacity)
  Current/1 -> SOCEstimator/2(Current)
  SOC_Initial/1 -> SOCEstimator/1(SOC_Initial)
  SOCEstimator/1(SOC) -> SOC/1

== system System3/Battery1/Module3/SubModule_2/Cell14/SOC_Mapping ==
  SOC : Inport
  Cell_Temp : Inport  Port=2
  2-D Lookup Table : Lookup_n-D  LookupTableObject=''  BreakpointsForDimension1Source=Input port  BreakpointsForDimension1=[0 0.1 0.2 0.3 0.4 0.5 0.6 0.7 0.8 0.9 1]  BreakpointsForDimension2=[0 10 20 30 40 50 60]  BreakpointsForDimension1FirstPoint=10  BreakpointsForDimension2FirstPoint=10  BreakpointsForDimension1Spacing=12  BreakpointsForDimension2Spacing=12  IndexSearchMethod=Evenly spaced points  TableSource=Input port  Table=|  InterpMethod=Akima spline  DiagnosticForOutOfRangeInput=Error  InternalRulePriority=Speed  RndMeth=Simplest
      | [
      |     2.954364, 3.109857, 3.273534, 3.3066, 3.34,    3.3734,  3.20473;
      |     3.122427, 3.286765, 3.459753, 3.4947, 3.53,    3.5653,  3.387035;
      |     3.175499, 3.342631, 3.518559, 3.5541, 3.59,    3.6259,  3.444605;
      |     3.210881, 3.379875, 3.557763, 3.5937, 3.63,    3.6663,  3.482985;
      |     3.237417, 3.407808, 3.587166, 3.6234, 3.66,    3.6966,  3.511777;
      |     3.272799, 3.445052, 3.62637,  3.663,  3.7,     3.737,   3.55015;
      |     3.317026, 3.491066, 3.675375, 3.7125, 3.75,    3.7875,  3.598125;
      |     3.387789, 3.566094, 3.753783, 3.7917, 3.83,    3.8683,  3.674885;
      |     3.467398, 3.649892, 3.841992, 3.8808, 3.92,    3.9592,  3.76124;
      |     3.564697, 3.752313, 3.949803, 3.9897, 4.03,    4.0703,  3.866785;
      |     3.653151, 3.845422, 4.047813, 4.0887, 4.13,    4.1713,  3.962735
      | ]
      settings: InputPortMap=u0,u1,p221,p5
  2-D Lookup Table1 : Lookup_n-D  LookupTableObject=''  BreakpointsForDimension1Source=Input port  BreakpointsForDimension1=[0 0.1 0.2 0.3 0.4 0.5 0.6 0.7 0.8 0.9 1]  BreakpointsForDimension2=[0 10 20 30 40 50 60]  BreakpointsForDimension1FirstPoint=10  BreakpointsForDimension2FirstPoint=10  BreakpointsForDimension1Spacing=12  BreakpointsForDimension2Spacing=12  IndexSearchMethod=Evenly spaced points  TableSource=Input port  Table=|  InterpMethod=Akima spline  DiagnosticForOutOfRangeInput=Error  InternalRulePriority=Speed  RndMeth=Simplest
      | [
      |     2.954364, 3.109857, 3.273534, 3.3066, 3.34,    3.3734,  3.20473;
      |     3.122427, 3.286765, 3.459753, 3.4947, 3.53,    3.5653,  3.387035;
      |     3.175499, 3.342631, 3.518559, 3.5541, 3.59,    3.6259,  3.444605;
      |     3.210881, 3.379875, 3.557763, 3.5937, 3.63,    3.6663,  3.482985;
      |     3.237417, 3.407808, 3.587166, 3.6234, 3.66,    3.6966,  3.511777;
      |     3.272799, 3.445052, 3.62637,  3.663,  3.7,     3.737,   3.55015;
      |     3.317026, 3.491066, 3.675375, 3.7125, 3.75,    3.7875,  3.598125;
      |     3.387789, 3.566094, 3.753783, 3.7917, 3.83,    3.8683,  3.674885;
      |     3.467398, 3.649892, 3.841992, 3.8808, 3.92,    3.9592,  3.76124;
      |     3.564697, 3.752313, 3.949803, 3.9897, 4.03,    4.0703,  3.866785;
      |     3.653151, 3.845422, 4.047813, 4.0887, 4.13,    4.1713,  3.962735
      | ]
      settings: InputPortMap=u0,u1,p221,p5
  Lookup Table Dynamic{3..6} (4 alike) : simulink/Lookup Tables/Lookup Table Dynamic  LookUpMeth=Interpolation-Use End Values  OutDataType=fixdt('double')  OutScaling=[]  OutputDataTypeScalingMode=Specify via dialog  OutDataTypeStr=fixdt('double')  DoSatur=off
  Ri : Outport
  R1 : Outport  Port=2
  C1 : Outport  Port=3
  R2 : Outport  Port=4
  C2 : Outport  Port=5
  OCV : Outport  Port=6
  wires:
  Cell_Temp/1 -> 2-D Lookup Table/2, 2-D Lookup Table1/2
  Lookup Table Dynamic6/1 -> C2/1
  [C2_User] -> Lookup Table Dynamic6/3
  Lookup Table Dynamic5/1 -> R2/1
  [R2_User] -> Lookup Table Dynamic5/3
  Lookup Table Dynamic4/1 -> C1/1
  [C1_User] -> Lookup Table Dynamic4/3
  Lookup Table Dynamic3/1 -> R1/1
  [R1_User] -> Lookup Table Dynamic3/3
  2-D Lookup Table1/1 -> Ri/1
  [Ri_User] -> 2-D Lookup Table1/3
  2-D Lookup Table/1 -> OCV/1
  [OCV] -> 2-D Lookup Table/3
  [SOC_User] -> 2-D Lookup Table1/4, Lookup Table Dynamic3/2, Lookup Table Dynamic4/2, Lookup Table Dynamic5/2, Lookup Table Dynamic6/2, 2-D Lookup Table/4
  SOC/1 -> 2-D Lookup Table/1, 2-D Lookup Table1/1, Lookup Table Dynamic4/1, Lookup Table Dynamic5/1, Lookup Table Dynamic6/1, Lookup Table Dynamic3/1

== system System3/Battery1/Module3/SubModule_2/Cell14/Subsystem ==
  Cell_Current : Inport
  Ri : Inport  Port=2
  Add : Sum  Inputs=+-
  Add1 : Sum  Inputs=-+
  Delay : Delay  DelayLength=1  InitialConditionSource=Input port
      settings: InputPortMap=u0,p4
  Divide : Product  Inputs=*/
  From3 : From  TagVisibility=global
  Integrator : Integrator  InitialConditionSource=external
  Product{,1..3} (4 alike) : Product
  Temp_Cell : Outport
  wires:
  [Cp] -> Divide/2
  Delay/1 -> Add/1
  [Temp_Iinitial] -> Integrator/2, Delay/2
  Divide/1 -> Integrator/1
  Add1/1 -> Divide/1
  Product1/1 -> Add1/2
  Product3/1 -> Add1/1
  Add/1 -> Product3/1
  [Temp_ambient] -> Add/2
  Product2/1 -> Product3/2
  From3/1 -> Product2/2
  [h] -> Product2/1
  Ri/1 -> Product1/2
  Product/1 -> Product1/1
  Cell_Current/1 -> Product/1, Product/2
  Integrator/1 -> Delay/1, Temp_Cell/1

== system System3/Battery1/Module3/SubModule_2/Cell15/2RC ==
  Current : Inport
  Ri : Inport  Port=2
  R1 : Inport  Port=3
  C1 : Inport  Port=4
  R2 : Inport  Port=5
  C2 : Inport  Port=6
  RC1 : Subsystem
  RC2 : Subsystem
  Rint : Subsystem
  V1 : Outport
  V2 : Outport  Port=2
  Vi : Outport  Port=3
  wires:
  Ri/1 -> Rint/2(R)
  C2/1 -> RC2/3(C)
  RC2/1(V) -> V2/1
  RC1/1(V) -> V1/1
  R2/1 -> RC2/2(R)
  C1/1 -> RC1/3(C)
  Rint/1(V) -> Vi/1
  R1/1 -> RC1/2(R)
  Current/1 -> RC2/1(Current), RC1/1(Current), Rint/1(Current)

== system System3/Battery1/Module3/SubModule_2/Cell15/SOCEstimator ==
  SOC_Initial : Inport
  Current : Inport  Port=2
  Cell_Capacity : Inport  Port=3
  SOCEstimator : Subsystem
  SOC : Outport
  wires:
  Cell_Capacity/1 -> SOCEstimator/3(CellCapacity)
  Current/1 -> SOCEstimator/2(Current)
  SOC_Initial/1 -> SOCEstimator/1(SOC_Initial)
  SOCEstimator/1(SOC) -> SOC/1

== system System3/Battery1/Module3/SubModule_2/Cell15/SOC_Mapping ==
  SOC : Inport
  Cell_Temp : Inport  Port=2
  2-D Lookup Table : Lookup_n-D  LookupTableObject=''  BreakpointsForDimension1Source=Input port  BreakpointsForDimension1=[0 0.1 0.2 0.3 0.4 0.5 0.6 0.7 0.8 0.9 1]  BreakpointsForDimension2=[0 10 20 30 40 50 60]  BreakpointsForDimension1FirstPoint=10  BreakpointsForDimension2FirstPoint=10  BreakpointsForDimension1Spacing=12  BreakpointsForDimension2Spacing=12  IndexSearchMethod=Evenly spaced points  TableSource=Input port  Table=|  InterpMethod=Akima spline  DiagnosticForOutOfRangeInput=Error  InternalRulePriority=Speed  RndMeth=Simplest
      | [
      |     2.954364, 3.109857, 3.273534, 3.3066, 3.34,    3.3734,  3.20473;
      |     3.122427, 3.286765, 3.459753, 3.4947, 3.53,    3.5653,  3.387035;
      |     3.175499, 3.342631, 3.518559, 3.5541, 3.59,    3.6259,  3.444605;
      |     3.210881, 3.379875, 3.557763, 3.5937, 3.63,    3.6663,  3.482985;
      |     3.237417, 3.407808, 3.587166, 3.6234, 3.66,    3.6966,  3.511777;
      |     3.272799, 3.445052, 3.62637,  3.663,  3.7,     3.737,   3.55015;
      |     3.317026, 3.491066, 3.675375, 3.7125, 3.75,    3.7875,  3.598125;
      |     3.387789, 3.566094, 3.753783, 3.7917, 3.83,    3.8683,  3.674885;
      |     3.467398, 3.649892, 3.841992, 3.8808, 3.92,    3.9592,  3.76124;
      |     3.564697, 3.752313, 3.949803, 3.9897, 4.03,    4.0703,  3.866785;
      |     3.653151, 3.845422, 4.047813, 4.0887, 4.13,    4.1713,  3.962735
      | ]
      settings: InputPortMap=u0,u1,p221,p5
  2-D Lookup Table1 : Lookup_n-D  LookupTableObject=''  BreakpointsForDimension1Source=Input port  BreakpointsForDimension1=[0 0.1 0.2 0.3 0.4 0.5 0.6 0.7 0.8 0.9 1]  BreakpointsForDimension2=[0 10 20 30 40 50 60]  BreakpointsForDimension1FirstPoint=10  BreakpointsForDimension2FirstPoint=10  BreakpointsForDimension1Spacing=12  BreakpointsForDimension2Spacing=12  IndexSearchMethod=Evenly spaced points  TableSource=Input port  Table=|  InterpMethod=Akima spline  DiagnosticForOutOfRangeInput=Error  InternalRulePriority=Speed  RndMeth=Simplest
      | [
      |     2.954364, 3.109857, 3.273534, 3.3066, 3.34,    3.3734,  3.20473;
      |     3.122427, 3.286765, 3.459753, 3.4947, 3.53,    3.5653,  3.387035;
      |     3.175499, 3.342631, 3.518559, 3.5541, 3.59,    3.6259,  3.444605;
      |     3.210881, 3.379875, 3.557763, 3.5937, 3.63,    3.6663,  3.482985;
      |     3.237417, 3.407808, 3.587166, 3.6234, 3.66,    3.6966,  3.511777;
      |     3.272799, 3.445052, 3.62637,  3.663,  3.7,     3.737,   3.55015;
      |     3.317026, 3.491066, 3.675375, 3.7125, 3.75,    3.7875,  3.598125;
      |     3.387789, 3.566094, 3.753783, 3.7917, 3.83,    3.8683,  3.674885;
      |     3.467398, 3.649892, 3.841992, 3.8808, 3.92,    3.9592,  3.76124;
      |     3.564697, 3.752313, 3.949803, 3.9897, 4.03,    4.0703,  3.866785;
      |     3.653151, 3.845422, 4.047813, 4.0887, 4.13,    4.1713,  3.962735
      | ]
      settings: InputPortMap=u0,u1,p221,p5
  Lookup Table Dynamic{3..6} (4 alike) : simulink/Lookup Tables/Lookup Table Dynamic  LookUpMeth=Interpolation-Use End Values  OutDataType=fixdt('double')  OutScaling=[]  OutputDataTypeScalingMode=Specify via dialog  OutDataTypeStr=fixdt('double')  DoSatur=off
  Ri : Outport
  R1 : Outport  Port=2
  C1 : Outport  Port=3
  R2 : Outport  Port=4
  C2 : Outport  Port=5
  OCV : Outport  Port=6
  wires:
  Cell_Temp/1 -> 2-D Lookup Table/2, 2-D Lookup Table1/2
  Lookup Table Dynamic6/1 -> C2/1
  [C2_User] -> Lookup Table Dynamic6/3
  Lookup Table Dynamic5/1 -> R2/1
  [R2_User] -> Lookup Table Dynamic5/3
  Lookup Table Dynamic4/1 -> C1/1
  [C1_User] -> Lookup Table Dynamic4/3
  Lookup Table Dynamic3/1 -> R1/1
  [R1_User] -> Lookup Table Dynamic3/3
  2-D Lookup Table1/1 -> Ri/1
  [Ri_User] -> 2-D Lookup Table1/3
  2-D Lookup Table/1 -> OCV/1
  [OCV] -> 2-D Lookup Table/3
  [SOC_User] -> 2-D Lookup Table1/4, Lookup Table Dynamic3/2, Lookup Table Dynamic4/2, Lookup Table Dynamic5/2, Lookup Table Dynamic6/2, 2-D Lookup Table/4
  SOC/1 -> 2-D Lookup Table/1, 2-D Lookup Table1/1, Lookup Table Dynamic4/1, Lookup Table Dynamic5/1, Lookup Table Dynamic6/1, Lookup Table Dynamic3/1

== system System3/Battery1/Module3/SubModule_2/Cell15/Subsystem ==
  Cell_Current : Inport
  Ri : Inport  Port=2
  Add : Sum  Inputs=+-
  Add1 : Sum  Inputs=-+
  Delay : Delay  DelayLength=1  InitialConditionSource=Input port
      settings: InputPortMap=u0,p4
  Divide : Product  Inputs=*/
  From3 : From  TagVisibility=global
  Integrator : Integrator  InitialConditionSource=external
  Product{,1..3} (4 alike) : Product
  Temp_Cell : Outport
  wires:
  [Cp] -> Divide/2
  Delay/1 -> Add/1
  [Temp_Iinitial] -> Integrator/2, Delay/2
  Divide/1 -> Integrator/1
  Add1/1 -> Divide/1
  Product1/1 -> Add1/2
  Product3/1 -> Add1/1
  Add/1 -> Product3/1
  [Temp_ambient] -> Add/2
  Product2/1 -> Product3/2
  From3/1 -> Product2/2
  [h] -> Product2/1
  Ri/1 -> Product1/2
  Product/1 -> Product1/1
  Cell_Current/1 -> Product/1, Product/2
  Integrator/1 -> Delay/1, Temp_Cell/1

== system System3/Battery1/Module3/SubModule_2/Cell16/2RC ==
  Current : Inport
  Ri : Inport  Port=2
  R1 : Inport  Port=3
  C1 : Inport  Port=4
  R2 : Inport  Port=5
  C2 : Inport  Port=6
  RC1 : Subsystem
  RC2 : Subsystem
  Rint : Subsystem
  V1 : Outport
  V2 : Outport  Port=2
  Vi : Outport  Port=3
  wires:
  Ri/1 -> Rint/2(R)
  C2/1 -> RC2/3(C)
  RC2/1(V) -> V2/1
  RC1/1(V) -> V1/1
  R2/1 -> RC2/2(R)
  C1/1 -> RC1/3(C)
  Rint/1(V) -> Vi/1
  R1/1 -> RC1/2(R)
  Current/1 -> RC2/1(Current), RC1/1(Current), Rint/1(Current)

== system System3/Battery1/Module3/SubModule_2/Cell16/SOCEstimator ==
  SOC_Initial : Inport
  Current : Inport  Port=2
  Cell_Capacity : Inport  Port=3
  SOCEstimator : Subsystem
  SOC : Outport
  wires:
  Cell_Capacity/1 -> SOCEstimator/3(CellCapacity)
  Current/1 -> SOCEstimator/2(Current)
  SOC_Initial/1 -> SOCEstimator/1(SOC_Initial)
  SOCEstimator/1(SOC) -> SOC/1
